simulink model "sim_battery_wo_cap"  (R2021a)
settings: Solver=VariableStepAuto  StartTime=0.0  StopTime=t_sim  RelTol=1e-3
values from neighbouring files (symbols this model uses):
  a = (phi'*phi)\phi'*u_oc    [init_script.m]    (also in sim_with_cap.m = block.DialogPrm(3).Data; sim_wo_cap.m = block.DialogPrm(2).data; sim_wo_cap_disc.m = block.DialogPrm(2).data)
  Delta = 0.04    [init_script.m]    (also in sim_with_cap.m = block.DialogPrm(1).Data; sim_wo_cap_disc.m = block.DialogPrm(4).data)
  Qe = 2.9*3600    (= 10440)    [init_script.m]    (also in sim_with_cap.m = block.DialogPrm(4).Data; sim_wo_cap.m = block.DialogPrm(3).data; sim_wo_cap_disc.m = block.DialogPrm(3).data)
  R0 = 0.75e3    (= 750)    [init_script.m]
  Rp = 1.8e3    (= 1800)    [init_script.m]
  soc0 = 0.3    [init_script.m]
libraries: fl_lib x6, nesl_utility x6, ee_lib x3
settings Model: Creator=saleh  LastModifiedBy=saleh

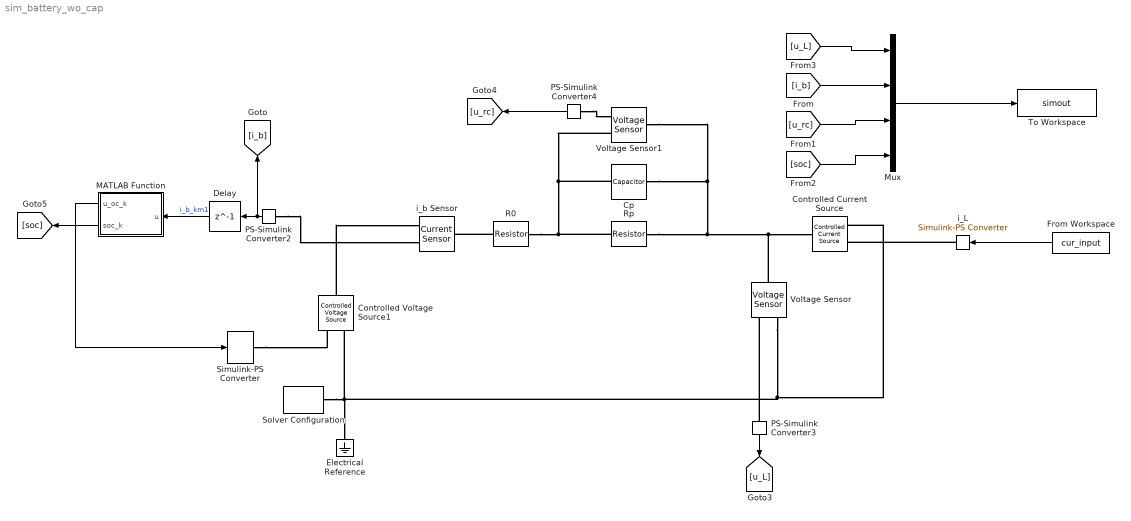
== system sim_battery_wo_cap ==
  Controlled Current Source : fl_lib/Electrical/Electrical Sources/Controlled Current Source
  Controlled Voltage Source1 : fl_lib/Electrical/Electrical Sources/Controlled Voltage Source
  Cp : ee_lib/Passive/Capacitor  cap_option=0  c=Cp F  Cvec=[1e-05, 1e-06] F  Vvec=[0, 10] V  CV_table_symmetry=1  f_vec=[1, 10] kHz  DFext_vec=[.8, 1.2]  C_tol=5  enable_C_tol=0  tol_distribution=1  nSigma=4  r=0 Ohm  g=0 1/Ohm  averaging_period=0 s  enable_operating_limits=0  operating_limit_action=2  max_working_voltage_range=[-25, 25] V  power_rating=1 W  enable_faults=0  fault_action=1  Cscale_faulted=100  R_faulted=1e-3 Ohm  G_faulted=0 1/Ohm  tau_fault=1e-3 s  enable_temporal_fault=0  t_fault=1 s  enable_behavioral_fault=0  max_permissible_voltage_range=[-100, 100] V  t_fail_on_voltage=1 s  i_specify=off  i_priority=None  i=0 A  i_nominal_specify=off  i_nominal_unit=A  i_nominal_value=1  v_specify=off  v_priority=None  v=0 V  v_nominal_specify=off  v_nominal_unit=V  v_nominal_value=1  vc_specify=off  vc_priority=High  vc=0 V  vc_nominal_specify=off  vc_nominal_unit=V  vc_nominal_value=1
  Delay : Delay  DelayLength=1  SampleTime=Delta
  Electrical Reference : fl_lib/Electrical/Electrical Elements/Electrical Reference
  From Workspace : FromWorkspace  VariableName=cur_input  SampleTime=Delta
  MATLAB Function : MATLAB Function  TreatAsAtomicUnit=on  SystemSampleTime=Delta
  Mux : Mux
  PS-Simulink Converter2 : nesl_utility/PS-Simulink Converter  PhysicalDomain=network_engine_domain  SubClassName=ps_output  LeftPortType=input  RightPortType=output  PseudoPeriodic=off  Frequencies=[]  Unit=inherit  AffineConversion=off
      settings: SourceProductBaseCode=PW,SS
  PS-Simulink Converter3 : nesl_utility/PS-Simulink Converter  PhysicalDomain=network_engine_domain  SubClassName=ps_output  LeftPortType=input  RightPortType=output  PseudoPeriodic=off  Frequencies=[]  Unit=inherit  AffineConversion=off
      settings: SourceProductBaseCode=PW,SS
  PS-Simulink Converter4 : nesl_utility/PS-Simulink Converter  PhysicalDomain=network_engine_domain  SubClassName=ps_output  LeftPortType=input  RightPortType=output  PseudoPeriodic=off  Frequencies=[]  Unit=inherit  AffineConversion=off
      settings: SourceProductBaseCode=PW,SS
  R0 : ee_lib/Passive/Resistor  R=R0 Ohm  R_tol=5  enable_R_tol=0  tol_distribution=1  nSigma=4  enable_operating_limits=0  operating_limit_action=2  max_working_voltage=100 V  power_rating=1 W  enable_faults=0  fault_action=1  R_faulted=inf Ohm  enable_temporal_fault=0  t_fault=1 s  enable_behavioral_fault=0  max_permissible_current=1 A  t_fail_on_current=1 s  noise_mode=0  sample_time=1e-3 s  repeatability=1  auto_seed=2270032532  user_seed=0  Tdevice=25 degC  alpha=3.93e-3 1/K  Tmeas=25 degC  thermal_mass=100 J/K  power_derating_T1=70 degC  power_derating_T2=155 degC  operating_temperature_range_vec=[-50, 150] degC  temperature_specify=off  temperature_priority=High  temperature=298.15 K  temperature_nominal_specify=off  temperature_nominal_unit=K  temperature_nominal_value=1
  Rp : ee_lib/Passive/Resistor  R=Rp Ohm  R_tol=5  enable_R_tol=0  tol_distribution=1  nSigma=4  enable_operating_limits=0  operating_limit_action=2  max_working_voltage=100 V  power_rating=1 W  enable_faults=0  fault_action=1  R_faulted=inf Ohm  enable_temporal_fault=0  t_fault=1 s  enable_behavioral_fault=0  max_permissible_current=1 A  t_fail_on_current=1 s  noise_mode=0  sample_time=1e-3 s  repeatability=1  auto_seed=1336658428  user_seed=0  Tdevice=25 degC  alpha=3.93e-3 1/K  Tmeas=25 degC  thermal_mass=100 J/K  power_derating_T1=70 degC  power_derating_T2=155 degC  operating_temperature_range_vec=[-50, 150] degC  temperature_specify=off  temperature_priority=High  temperature=298.15 K  temperature_nominal_specify=off  temperature_nominal_unit=K  temperature_nominal_value=1
  Simulink-PS Converter : nesl_utility/Simulink-PS Converter  PhysicalDomain=network_engine_domain  SubClassName=ps_input  LeftPortType=input  RightPortType=output  PseudoPeriodic=off  Frequencies=[]  NoiseDistribution=none  NoiseParameters=[]  Unit=V  AffineConversion=off  FilteringAndDerivatives=provide  SimscapeFilterOrder=1  InputFilterTimeConstant=0.001  UdotUserProvided=0
      settings: SourceProductBaseCode=PW,SS
  Solver Configuration : nesl_utility/Solver Configuration  PhysicalDomain=network_engine_domain  SubClassName=solver  LeftPortType=input  RightPortType=generic  Tones=[]  Harmonics=[]  SimulateNoise=off  Profile=off  UseLocalSampling=off  EnableSwitchedLinearOptims=on  FrequencyDomain=off  UseCCode=off  RelTol=0.001  AbsTol=1e-06  MinStep=1e-09  ToWorkspace=off  RevertToSquareIcSolve=off  NumHomotopyIterations=100  PhasorMode=off  PhasorModeNumHarmonics=1  DoDC=off  ResidualTolerance=1e-09  UseLocalSolver=off  LocalSolverChoice=NE_BACKWARD_EULER_ADVANCER  LocalSolverSampleTime=0.001  DoFixedCost=off  MaxNonlinIter=3  MaxModeIter=2  ComputeImpulses=off  ImpulseIterations=2  LinearAlgebra=auto  EquationFormulation=NE_TIME_EF  DelaysMemoryBudget=1024  AutomaticFiltering=on  FilteringTimeConstant=0.001  PartitionStorageMethod=AS_NEEDED  PartitionMemoryBudget=1024  PartitionMethod=ROBUST
      settings: SourceProductBaseCode=PW,SS
  To Workspace : ToWorkspace  VariableName=simout  SampleTime=-1
  Voltage Sensor : fl_lib/Electrical/Electrical Sensors/Voltage Sensor
  Voltage Sensor1 : fl_lib/Electrical/Electrical Sensors/Voltage Sensor
  i_L : nesl_utility/Simulink-PS Converter  PhysicalDomain=network_engine_domain  SubClassName=ps_input  LeftPortType=input  RightPortType=output  PseudoPeriodic=off  Frequencies=[]  NoiseDistribution=none  NoiseParameters=[]  Unit=A  AffineConversion=off  FilteringAndDerivatives=provide  SimscapeFilterOrder=1  InputFilterTimeConstant=0.001  UdotUserProvided=0
      settings: SourceProductBaseCode=PW,SS
  i_b Sensor : fl_lib/Electrical/Electrical Sensors/Current Sensor
  wires:
  Mux/1 -> To Workspace/1
  [soc] -> Mux/4
  [u_L] -> Mux/1
  [u_rc] -> Mux/3
  PS-Simulink Converter3/1 -> [u_L]
  PS-Simulink Converter4/1 -> [u_rc]
  [i_b] -> Mux/2
  From Workspace/1 -> i_L/1
  MATLAB Function/1(u_oc_k) -> Simulink-PS Converter/1
  PS-Simulink Converter2/1 -> Delay/1, [i_b]
  MATLAB Function/2(soc_k) -> [soc]
  Delay/1 -> MATLAB Function/1(u)  "i_b_km1"
  connections:
  Controlled Voltage Source1/RConn2 -- Electrical Reference/LConn1 -- Controlled Current Source/RConn2 -- Voltage Sensor/RConn2 -- Solver Configuration/RConn1
  Voltage Sensor1/LConn1 -- Cp/LConn1 -- Rp/LConn1 -- Voltage Sensor/LConn1 -- Controlled Current Source/LConn1
  Cp/RConn1 -- Voltage Sensor1/RConn2 -- R0/LConn1 -- Rp/RConn1
  PS-Simulink Converter2/LConn1 -- i_b Sensor/RConn1
  PS-Simulink Converter3/LConn1 -- Voltage Sensor/RConn1
  R0/RConn1 -- i_b Sensor/LConn1
  Controlled Voltage Source1/LConn1 -- i_b Sensor/RConn2
  PS-Simulink Converter4/LConn1 -- Voltage Sensor1/RConn1
  i_L/RConn1 -- Controlled Current Source/RConn1
  Simulink-PS Converter/RConn1 -- Controlled Voltage Source1/RConn1

== matlab function sim_battery_wo_cap/MATLAB Function ==
  data: u input; u_oc_k output; soc_k output; soc0 parameter; Qe parameter; Delta parameter; a parameter
function [u_oc_k, soc_k] = fcn(u, soc0, Qe, Delta, a)

persistent soc
if isempty(soc)
    soc = soc0;
end
soc = soc + Delta*u/Qe;
u_oc_k = a(1)*soc^2 + a(2)*soc + a(3);
soc_k = soc;
